simulink model "PMSM_Only_Equations"  (R2017b)
settings: Solver=ode15s  StartTime=0.0  StopTime=1  FixedStep=0.0001  RelTol=1e-3
InitFcn:
  | r=1.2
  | Ld=5.7*10^-3
  | Lq=12.5*10^-3
  | PM=123*10^-3
  | P=4
  | b=0
  | J=0.0001
settings Model: Creator=Aliraqe  LastModifiedBy=Aliraqe

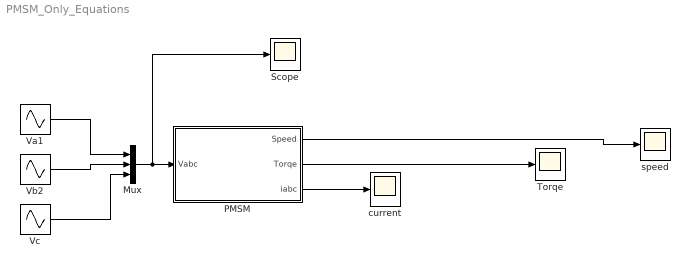
== system PMSM_Only_Equations ==
  Mux : Mux  Inputs=3
  PMSM : Subsystem
  Scope : Scope
  "Torqe " : Scope
  Va1 : Sin  Amplitude=257  Frequency=2*pi*60  SampleTime=0.0001
  Vb2 : Sin  Amplitude=257  Frequency=2*pi*60  Phase=-2*pi/3  SampleTime=0.0001
  Vc : Sin  Amplitude=257  Frequency=2*pi*60  Phase=2*pi/3  SampleTime=0.0001
  current : Scope
  speed : Scope
  wires:
  Mux/1 -> Scope/1, PMSM/1(Vabc)
  PMSM/1("Speed ") -> speed/1
  PMSM/2(Torqe) -> "Torqe "/1
  PMSM/3(iabc) -> current/1
  Vc/1 -> Mux/3
  Vb2/1 -> Mux/2
  Va1/1 -> Mux/1

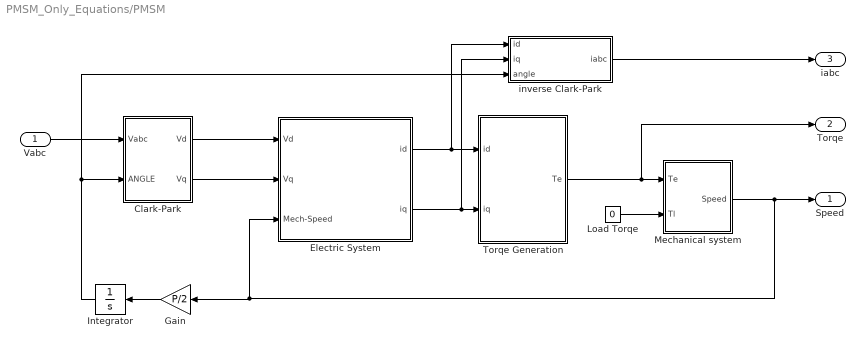
== system PMSM_Only_Equations/PMSM ==
  Vabc : Inport
  Clark-Park : Subsystem
  "Electric System " : Subsystem
  Gain : Gain  Gain=P/2
  Integrator : Integrator
  Load Torqe : Constant  Value=0
  Mechanical system : Subsystem
  Torqe Generation : Subsystem
  inverse Clark-Park : Subsystem
  "Speed " : Outport
  Torqe : Outport  Port=2
  iabc : Outport  Port=3
  wires:
  Load Torqe/1 -> Mechanical system/2(Tl)
  Clark-Park/1(Vd) -> "Electric System "/1(Vd)
  Torqe Generation/1(Te) -> Torqe/1, Mechanical system/1(Te)
  Clark-Park/2(Vq) -> "Electric System "/2("Vq ")
  Mechanical system/1(Speed) -> "Speed "/1, "Electric System "/3("Mech-Speed "), Gain/1
  "Electric System "/1("id ") -> Torqe Generation/1(id), inverse Clark-Park/1(id)
  Vabc/1 -> Clark-Park/1(Vabc)
  "Electric System "/2(iq) -> inverse Clark-Park/2(iq), Torqe Generation/2("iq ")
  Gain/1 -> Integrator/1
  Integrator/1 -> inverse Clark-Park/3(angle), Clark-Park/2("ANGLE ")
  inverse Clark-Park/1(iabc) -> iabc/1

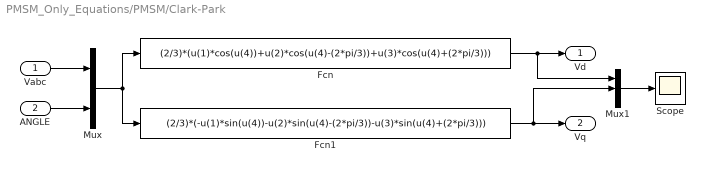
== system PMSM_Only_Equations/PMSM/Clark-Park ==
  Vabc : Inport
  "ANGLE " : Inport  Port=2
  Fcn : Fcn  Expr=(2/3)*(u(1)*cos(u(4))+u(2)*cos(u(4)-(2*pi/3))+u(3)*cos(u(4)+(2*pi/3)))
  Fcn1 : Fcn  Expr=(2/3)*(-u(1)*sin(u(4))-u(2)*sin(u(4)-(2*pi/3))-u(3)*sin(u(4)+(2*pi/3)))
  Mux : Mux  Inputs=2
  Mux1 : Mux  Inputs=3
  Scope : Scope
  Vd : Outport
  Vq : Outport  Port=2
  wires:
  Fcn/1 -> Mux1/1, Vd/1
  Vabc/1 -> Mux/1
  Mux/1 -> Fcn1/1, Fcn/1
  Fcn1/1 -> Mux1/2, Vq/1
  Mux1/1 -> Scope/1
  "ANGLE "/1 -> Mux/2

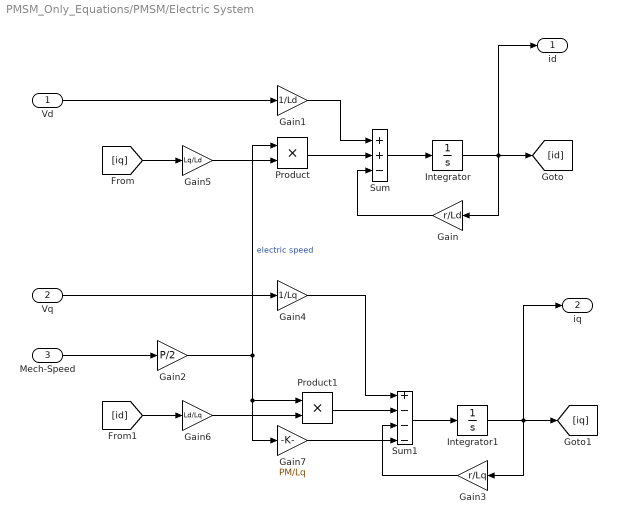
== system PMSM_Only_Equations/PMSM/Electric System  ==
  Vd : Inport
  "Vq " : Inport  Port=2
  "Mech-Speed " : Inport  Port=3
  Gain : Gain  Gain=r/Ld
  Gain1 : Gain  Gain=1/Ld
  Gain2 : Gain  Gain=P/2
  Gain3 : Gain  Gain=r/Lq
  Gain4 : Gain  Gain=1/Lq
  Gain5 : Gain  Gain=Lq/Ld
  Gain6 : Gain  Gain=Ld/Lq
  Gain7 : Gain  Gain=PM/Lq
  Integrator : Integrator
  Integrator1 : Integrator
  Product : Product
  Product1 : Product
  Sum : Sum  Inputs=++-
  Sum1 : Sum  Inputs=+---
  "id " : Outport
  iq : Outport  Port=2
  wires:
  Integrator/1 -> "id "/1, [id], Gain/1
  Gain1/1 -> Sum/1
  Sum/1 -> Integrator/1
  Vd/1 -> Gain1/1
  Gain/1 -> Sum/3
  Product/1 -> Sum/2
  Gain3/1 -> Sum1/3
  Gain4/1 -> Sum1/1
  Product1/1 -> Sum1/2
  "Vq "/1 -> Gain4/1
  Sum1/1 -> Integrator1/1
  Integrator1/1 -> iq/1, [iq], Gain3/1
  "Mech-Speed "/1 -> Gain2/1
  Gain2/1 -> Gain7/1, Product1/1, Product/1  "electric speed"
  [iq] -> Gain5/1
  Gain5/1 -> Product/2
  [id] -> Gain6/1
  Gain6/1 -> Product1/2
  Gain7/1 -> Sum1/4

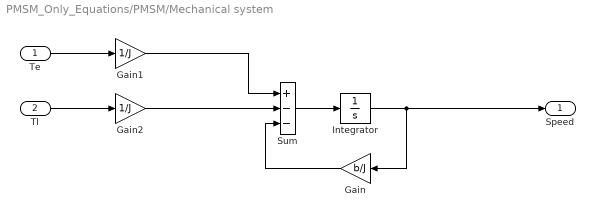
== system PMSM_Only_Equations/PMSM/Mechanical system ==
  Te : Inport
  Tl : Inport  Port=2
  Gain : Gain  Gain=b/J
  Gain1 : Gain  Gain=1/J
  Gain2 : Gain  Gain=1/J
  Integrator : Integrator
  Sum : Sum  Inputs=+--
  Speed : Outport
  wires:
  Integrator/1 -> Speed/1, Gain/1
  Gain1/1 -> Sum/1
  Gain2/1 -> Sum/2
  Sum/1 -> Integrator/1
  Gain/1 -> Sum/3
  Te/1 -> Gain1/1
  Tl/1 -> Gain2/1

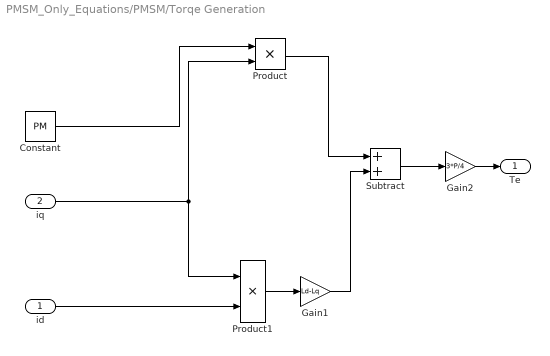
== system PMSM_Only_Equations/PMSM/Torqe Generation ==
  id : Inport
  "iq " : Inport  Port=2
  Constant : Constant  Value=PM
  Gain1 : Gain  Gain=Ld-Lq
  Gain2 : Gain  Gain=3*P/4
  Product : Product
  Product1 : Product
  Subtract : Sum
  Te : Outport
  wires:
  id/1 -> Product1/2
  Constant/1 -> Product/1
  "iq "/1 -> Product1/1, Product/2
  Product/1 -> Subtract/1
  Subtract/1 -> Gain2/1
  Gain2/1 -> Te/1
  Product1/1 -> Gain1/1
  Gain1/1 -> Subtract/2

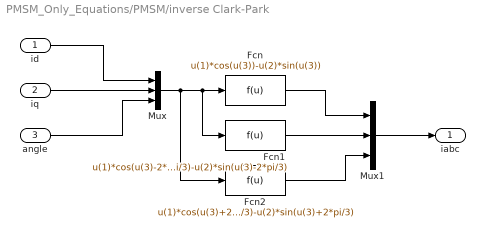
== system PMSM_Only_Equations/PMSM/inverse Clark-Park ==
  id : Inport
  iq : Inport  Port=2
  angle : Inport  Port=3
  Fcn : Fcn  Expr=u(1)*cos(u(3))-u(2)*sin(u(3))
  Fcn1 : Fcn  Expr=u(1)*cos(u(3)-2*pi/3)-u(2)*sin(u(3)-2*pi/3)
  Fcn2 : Fcn  Expr=u(1)*cos(u(3)+2*pi/3)-u(2)*sin(u(3)+2*pi/3)
  Mux : Mux  Inputs=3
  Mux1 : Mux  Inputs=3
  iabc : Outport
  wires:
  id/1 -> Mux/1
  iq/1 -> Mux/2
  angle/1 -> Mux/3
  Mux/1 -> Fcn2/1, Fcn1/1, Fcn/1
  Fcn/1 -> Mux1/1
  Fcn1/1 -> Mux1/2
  Fcn2/1 -> Mux1/3
  Mux1/1 -> iabc/1
